simulink model "DrivetrainEv"  (R2017b)
settings: Solver=VariableStepAuto  StartTime=0.0  StopTime=inf  RelTol=1e-3  EnableMultiTasking=on
model workspace (MAT data in the model file):
  Af = 2.27
  Bx = 10
  Cd = 0.28
  Cl = 0.1
  Cpm = 0.1
  Cx = 1.65
  Dx = 1
  Ex = 0.01
  FZMAX = 6570
  FZMIN = 0
  FsbF = [-700000 -7000 -700 0 700 7000 700000]
  FsbR = [-700000 -7000 -700 0 700 7000 700000]
  FskF = [-8928.57142857 -178.571428571 0 357.142857143 535.714285714 9285.71428571]
  FskR = [-5357.14285714 -107.142857143 0 214.285714286 321.428571429 5571.42857143]
  Iyy = 3000
  Iyy_Whl = 0.8
  Jd = 0.025
  Jmotor = 0.1
  Jw1 = 0.01
  Jw2 = 0.01
  Lrel = 0.15
  Mass = 1500
  NF = 2
  NR = 2
  Ndiff = 7.94
  Pabs = 101325
  Re = 0.327
  Rm = 0.15
  T = 273
  UNLOADED_RADIUS = 0.336
  VXLOW = 2
  aMy = 0.01
  a_CG = 1.188
  alphaMy = 0
  b = Simulink.Parameter
  b.Value = 100
  b.DataType = 'auto'
  b.Dimensions = [1 1]
  bMy = 0
  b_CG = 1.512
  bd = 0.001
  betaMy = 1
  br = 0.001
  bw1 = 0.001
  bw2 = 0.001
  cMy = 0
  disk_abore = 0.05
  domega_o = 0
  dzdotsF = [-10 -1 -0.1 0 0.1 1 10]
  dzdotsR = [-10 -1 -0.1 0 0.1 1 10]
  dzsF = [-0.005 -0.0001 0 0.2 0.2001 0.2051]
  dzsR = [-0.005 -0.0001 0 0.2 0.2001 0.2051]
  g = 9.81
  h = 0.5
  k = Simulink.Parameter
  k.Value = 5000
  k.DataType = 'auto'
  k.Dimensions = [1 1]
  kappamax = 1.5
  lam_x = 1
  mu_kinetic = 0.35
  mu_static = 0.45
  num_pads = 2
  omega_c = Simulink.Parameter
  omega_c.Value = 100
  omega_c.DataType = 'auto'
  omega_c.Dimensions = [1 1]
  omega_o = 0
  omegao = 0
  omegaw1o = 0
  omegaw2o = 0
  press = 234400
  q_o = 0
  theta_o = 0
  theta_o_Veh = 0
  wc_shaft = Simulink.Parameter
  wc_shaft.Value = 0.1
  wc_shaft.DataType = 'auto'
  wc_shaft.Dimensions = [1 1]
  x_o = 0
  xdot_o = 0
  z_o = -0.35
  zdot_o = 0
libraries: autolibsharedcoupling x3, autolibshared x3, autolibshareddiff x1
(part 1 of 2)
settings Model: ModifiedByFormat=The MathWorks, Inc.  SimulationMode=accelerator  PauseTimes=10  Creator=The MathWorks, Inc.  LastModifiedBy=The MathWorks, Inc.
settings DataIOCC: DSMLogging=off
settings DebuggingCC: UnderspecifiedInitializationDetection=Classic  MergeDetectMultiDrivingBlocksExec=none
settings ModelReferenceCC: PropagateSignalLabelsOutOfModel=off
settings CodeAppCC: StateflowObjectComments=on
settings GRTTargetCC: TargetLangStandard=C89/C90 (ANSI)
settings ConfigComp: CovMetricSettings=dsw  CovHtmlReporting=on  CovSaveCumulativeToWorkspaceVar=on  CovSaveSingleToWorkspaceVar=on  CovShowResultsExplorer=off  CovExternalEMLEnable=off
settings SimscapeCC: SimscapeNormalizeSystem=off

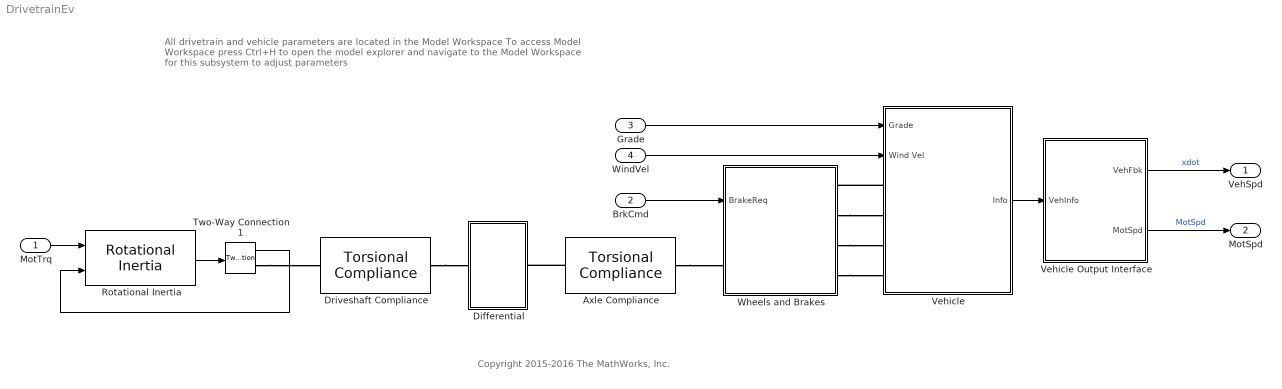
== system DrivetrainEv ==
  note: Copyright 2015-2016 The MathWorks, Inc.
  note: All drivetrain and vehicle parameters are located in the Model Workspace
      | To access Model Workspace press Ctrl+H to open the model explorer and navigate to the Model Workspace for this subsystem to adjust parameters
  MotTrq : Inport
  BrkCmd : Inport  Port=2
  Grade : Inport  Port=3
  WindVel : Inport  Port=4
  Axle Compliance : autolibsharedcoupling/Torsional Compliance  port_config=Two-way connection  k=k  b=b  theta_o=theta_o  domega_o=domega_o  omega_c=omega_c  blkID=0
      settings: SourceProductName=Powertrain Blockset  SourceProductBaseCode=PW
  Differential : Subsystem
  Driveshaft Compliance : autolibsharedcoupling/Torsional Compliance  port_config=Two-way connection  k=k  b=b  theta_o=theta_o  domega_o=domega_o  omega_c=omega_c  blkID=0
      settings: SourceProductName=Powertrain Blockset  SourceProductBaseCode=PW
  Rotational Inertia : autolibsharedcoupling/Rotational Inertia  port_config=Simulink  J=Jmotor  b=.001  omega_o=omega_o  externJ=off  blkID=0
      settings: SourceProductName=Powertrain Blockset  SourceProductBaseCode=PW
  Two-Way Connection1 : TwoWayConnection
  Vehicle : Subsystem
  Vehicle Output Interface : Subsystem
  Wheels and Brakes : Subsystem
  VehSpd : Outport
  MotSpd : Outport  Port=2  BusOutputAsStruct=on
  wires:
  BrkCmd/1 -> Wheels and Brakes/1(BrakeReq)
  MotTrq/1 -> Rotational Inertia/1
  Vehicle/1(Info) -> Vehicle Output Interface/1(VehInfo)
  Vehicle Output Interface/1(VehFbk) -> VehSpd/1  "xdot"
  Vehicle Output Interface/2(MotSpd) -> MotSpd/1  "MotSpd"
  Two-Way Connection1/1 -> Rotational Inertia/2
  Rotational Inertia/1 -> Two-Way Connection1/1
  WindVel/1 -> Vehicle/2(Wind Vel)
  Grade/1 -> Vehicle/1(Grade)
  connections:
  Wheels and Brakes/RConn2 -- Vehicle/LConn2
  Vehicle/LConn1 -- Wheels and Brakes/RConn1
  Wheels and Brakes/RConn4 -- Vehicle/LConn4
  Wheels and Brakes/RConn3 -- Vehicle/LConn3
  Axle Compliance/RConn1 -- Wheels and Brakes/LConn1
  Axle Compliance/LConn1 -- Differential/RConn1
  Driveshaft Compliance/RConn1 -- Differential/LConn1
  Two-Way Connection1/RConn1 -- Driveshaft Compliance/LConn1

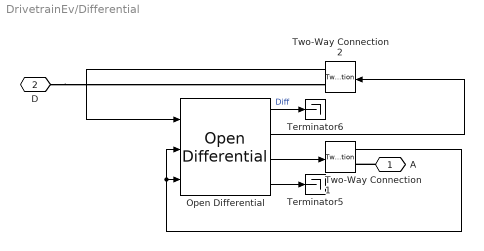
== system DrivetrainEv/Differential ==
  Open Differential : autolibshareddiff/Open Differential  shaftSwitchMask=To the left of center-line  Ndiff=Ndiff  Jd=Jd  bd=bd  Jw1=Jw1  bw1=bw1  Jw2=Jw2  bw2=bw2  omegaw1o=omegaw1o  omegaw2o=omegaw2o  maxAbsSpd=5e3
      settings: SourceProductName=Powertrain Blockset
  Terminator5 : Terminator
  Terminator6 : Terminator
  Two-Way Connection1 : TwoWayConnection
  Two-Way Connection2 : TwoWayConnection
  A : PMIOPort  Port=1  Side=Right
  D : PMIOPort  Port=2  Side=Left
  wires:
  Open Differential/3 -> Two-Way Connection1/1
  Open Differential/4 -> Terminator5/1
  Open Differential/1 -> Terminator6/1  "Diff"
  Open Differential/2 -> Two-Way Connection2/1
  Two-Way Connection1/1 -> Open Differential/3, Open Differential/2
  Two-Way Connection2/1 -> Open Differential/1
  connections:
  A/RConn1 -- Two-Way Connection1/RConn1
  D/RConn1 -- Two-Way Connection2/RConn1

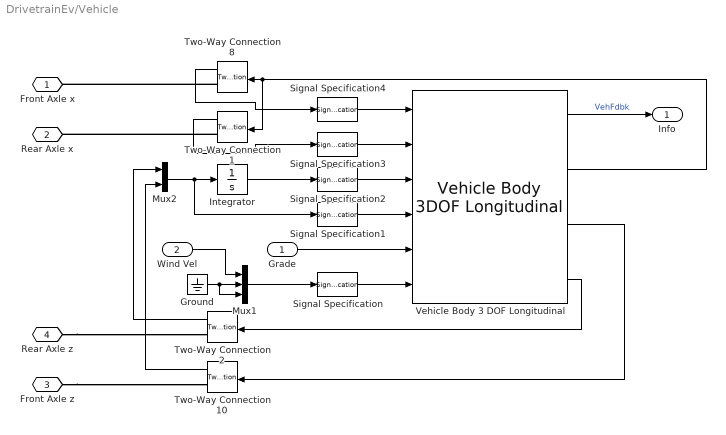
== system DrivetrainEv/Vehicle ==
  Grade : Inport  Unit=deg
  Wind Vel : Inport  Port=2  Unit=m/s
  Ground : Ground
  Integrator : Integrator
  Mux1 : Mux  Inputs=3
  Mux2 : Mux  Inputs=2
  Signal Specification : SignalSpecification  Unit=m/s
  Signal Specification1 : SignalSpecification  Unit=m/s
  Signal Specification2 : SignalSpecification  Unit=m
  Signal Specification3 : SignalSpecification  Unit=N
  Signal Specification4 : SignalSpecification  Unit=N
  Two-Way Connection{1..2,8,10} (4 alike) : TwoWayConnection
  Vehicle Body 3 DOF Longitudinal : autolibshared/Vehicle Body 3DOF Longitudinal  VariantControl=SL  groundType=Axle displacement, velocity  NF=NF  NR=NR  m=Mass  a=a_CG  b=b_CG  h=h  Cd=Cd  Af=Af  x_o=x_o  xdot_o=xdot_o  Cl=Cl  z_o=z_o  zdot_o=zdot_o  Iyy=Iyy  Cpm=Cpm  theta_o=theta_o_Veh  q_o=q_o  FskF=FskF  dzsF=dzsF  FsbF=FsbF  dzdotsF=dzdotsF  FskR=FskR  dzsR=dzsR  FsbR=FsbR  dzdotsR=dzdotsR  Pabs=Pabs  T=T  g=g  blkID=0
      settings: SourceProductName=Powertrain Blockset  SourceProductBaseCode=PW
  Front Axle x : PMIOPort  Port=1  Side=Left
  Rear Axle x : PMIOPort  Port=2  Side=Left
  Front Axle z : PMIOPort  Port=3  Side=Left
  Rear Axle z : PMIOPort  Port=4  Side=Left
  Info : Outport
  wires:
  Vehicle Body 3 DOF Longitudinal/3 -> Two-Way Connection10/1
  Vehicle Body 3 DOF Longitudinal/2 -> Two-Way Connection1/1, Two-Way Connection8/1
  Two-Way Connection8/1 -> Signal Specification4/1
  Vehicle Body 3 DOF Longitudinal/1 -> Info/1  "VehFdbk"
  Ground/1 -> Mux1/2, Mux1/3
  Mux1/1 -> Signal Specification/1
  Two-Way Connection1/1 -> Signal Specification3/1
  Vehicle Body 3 DOF Longitudinal/4 -> Two-Way Connection2/1
  Two-Way Connection2/1 -> Mux2/1
  Two-Way Connection10/1 -> Mux2/2
  Mux2/1 -> Integrator/1, Signal Specification1/1
  Integrator/1 -> Signal Specification2/1
  Wind Vel/1 -> Mux1/1
  Grade/1 -> Vehicle Body 3 DOF Longitudinal/5
  Signal Specification/1 -> Vehicle Body 3 DOF Longitudinal/6
  Signal Specification1/1 -> Vehicle Body 3 DOF Longitudinal/4
  Signal Specification2/1 -> Vehicle Body 3 DOF Longitudinal/3
  Signal Specification3/1 -> Vehicle Body 3 DOF Longitudinal/2
  Signal Specification4/1 -> Vehicle Body 3 DOF Longitudinal/1
  connections:
  Two-Way Connection8/RConn1 -- Front Axle x/RConn1
  Front Axle z/RConn1 -- Two-Way Connection10/RConn1
  Two-Way Connection1/RConn1 -- Rear Axle x/RConn1
  Rear Axle z/RConn1 -- Two-Way Connection2/RConn1

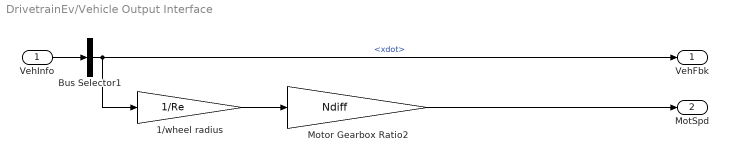
== system DrivetrainEv/Vehicle Output Interface ==
  VehInfo : Inport
  1/wheel radius : Gain  Gain=1/Re
  Bus Selector1 : BusSelector  OutputSignals=BdyFrm.Cg.Vel.xdot
  Motor Gearbox Ratio2 : Gain  Gain=Ndiff
  VehFbk : Outport
  MotSpd : Outport  Port=2
  wires:
  Bus Selector1/1 -> VehFbk/1, 1/wheel radius/1  "<xdot>"
  VehInfo/1 -> Bus Selector1/1
  1/wheel radius/1 -> Motor Gearbox Ratio2/1
  Motor Gearbox Ratio2/1 -> MotSpd/1
